simulink model "N3Z_tonetestError"  (R2014b)
settings: Solver=ode3  SolverMode=SingleTasking  StartTime=0.0  StopTime=1e-4  FixedStep=fpgaclk  RelTol=1e-3
PreLoadFcn:
  | %fpgaclk=1/32.768e6
  | fpgaclk=1/49.162e6
  | 
  | SerialData=[1,zeros(1,11),1,0,0,1]
  | load ../N3workingG/window
  | win=win';  %Go back to using flatter and wider windowed sync function
  | %load ../N3workingG/hanning    %use Hahn window
  | 
  | load ../N3workingG/PREemphasis   %For pre-empasis and deemphasis FIRs
  | 
  | %LUT3=xls2LUT2('../IQI_Qdemod.xls'); LUT3
  | load ../N3workingG/LUT3
  | load ../N3workingG/FIRiq2
  | % xls2LUT
  | 
  | GetProgFiles
  | 
  | PinAssignments    %Get Pin references for TE0722
  | 
  | 
  | 
  | 
  | 
  | %LCD
  | LCDdata=[LCD_D7,LCD_D6,LCD_D5,LCD_D4,LCD_D3,LCD_D2,LCD_D1,LCD_D0] %Note MSB...LSB!
  | LCDctrl=[LCD_E,LCD_RW,LCD_RS];
  | 
  | %for RS232 on pins 3 and 5 of USBB
  | 
  | %BT chip connections for WT12
  | 
  | RX_BT=RXD
  | TX_BT=TXD
  | 
  | RST_BB=RES
  | 
  | %PCMC=PCMC
  | %PCMS=PCMS
  | %PCMI=PCMI
  | %PCMO=PCMO
  | 
  | %Aliases:
  | SRDBT=PCMI
  | STDBT=PCMO
  | SCLK_BT=PCMC
  | SFS_BT=PCMS
  | 
  | %ADC control
  | 
  | %SDOA=SDOA
  | %SDOB=SDOB
  | %SCK=SCK
  | CONV=Csbar
  | CAL=Cal
  | 
  | ADC_G=[ADC_G3,ADC_G2,ADC_G1,ADC_G0]
  | %PD settings hard coded now
  | 
  | %%%%%%
  | TX_LOW=TX_Low
  | ... (+11 lines)
StartFcn:
  | SerialData=[1,zeros(1,11),1,0,0,1]
values from neighbouring files (symbols this model uses):
  ADC_G0 = {'P10'}    [PinAssignments.m]
  ADC_G1 = {'P11'}    [PinAssignments.m]
  ADC_G2 = {'N14'}    [PinAssignments.m]
  ADC_G3 = {'M11'}    [PinAssignments.m]
  Cal = {'L12'}    [PinAssignments.m]
  Csbar = {'M12'}    [PinAssignments.m]
  LCD_D0 = {'J13'}    [PinAssignments.m]
  LCD_D1 = {'J14'}    [PinAssignments.m]
  LCD_D2 = {'F15'}    [PinAssignments.m]
  LCD_D3 = {'H14'}    [PinAssignments.m]
  LCD_D4 = {'G12'}    [PinAssignments.m]
  LCD_D5 = {'L15'}    [PinAssignments.m]
  LCD_D6 = {'M14'}    [PinAssignments.m]
  LCD_D7 = {'K15'}    [PinAssignments.m]
  PCMC = {'H11'}    [PinAssignments.m]
  PCMI = {'H12'}    [PinAssignments.m]
  PCMO = {'N13'}    [PinAssignments.m]
  PCMS = {'M10'}    [PinAssignments.m]
  RES = {'G11'}    [PinAssignments.m]
  RXD = {'H13'}    [PinAssignments.m]
  TX_Low = {'P15'}    [PinAssignments.m]
  TXD = {'P13'}    [PinAssignments.m]
undefined symbols (not defined in the file or in its folder): AXI4, FIRRX, FIRTX, Lite
libraries: xbsIndex_r4 x1238, MyFunctions x43
(part 8 of 9)

== system N3Z_tonetestError/KeyPadinterface/OutputRegister/Subsystem5 ==
  Data : Inport
  PortId : Inport  Port=2
  Write : Inport  Port=3
  Logical : xbsIndex_r4/Logical  logical_function=AND  inputs=2  en=off  latency=0  precision=Full  arith_type=Unsigned  n_bits=8  bin_pt=2  align_bp=on  dbl_ovrd=off  block_type=logical
      settings: xl_area=[1 0 0 1 0 0 0]  block_version=VER_STRING_GOES_HERE
  PortAddress : xbsIndex_r4/Constant  const=3  gui_display_data_type=Fixed-point  arith_type=Unsigned  n_bits=8  bin_pt=0  preci_type=Single  exp_width=8  frac_width=24  explicit_period=on  period=fpgaclk  equ=P=C  opselect=C  inp2=PCIN>>17  opr=+  inp1=P  carry=CIN  dbl_ovrd=off  block_type=constant
      settings: block_version=VER_STRING_GOES_HERE
  Register1 : xbsIndex_r4/Register  init=0  rst=off  en=on  dbl_ovrd=off  block_type=register
      settings: xl_area=[4 8 0 0 0 0 0]  block_version=VER_STRING_GOES_HERE
  Relational1 : xbsIndex_r4/Relational  mode=a=b  op_type=Bool  en=off  latency=0  dbl_ovrd=off  block_type=relational
      settings: xl_area=[2 0 0 4 0 0 0]  block_version=VER_STRING_GOES_HERE
  LatchedData : Outport
  wires:
  Relational1/1 -> Logical/1
  Logical/1 -> Register1/2
  PortAddress/1 -> Relational1/2
  Data/1 -> Register1/1
  PortId/1 -> Relational1/1
  Write/1 -> Logical/2
  Register1/1 -> LatchedData/1

== system N3Z_tonetestError/KeyPadinterface/OutputRegister/Subsystem6 ==
  Data : Inport
  PortId : Inport  Port=2
  Write : Inport  Port=3
  Logical : xbsIndex_r4/Logical  logical_function=AND  inputs=2  en=off  latency=0  precision=Full  arith_type=Unsigned  n_bits=8  bin_pt=2  align_bp=on  dbl_ovrd=off  block_type=logical
      settings: xl_area=[1 0 0 1 0 0 0]  block_version=VER_STRING_GOES_HERE
  PortAddress : xbsIndex_r4/Constant  const=7  gui_display_data_type=Fixed-point  arith_type=Unsigned  n_bits=8  bin_pt=0  preci_type=Single  exp_width=8  frac_width=24  explicit_period=on  period=fpgaclk  equ=P=C  opselect=C  inp2=PCIN>>17  opr=+  inp1=P  carry=CIN  dbl_ovrd=off  block_type=constant
      settings: block_version=VER_STRING_GOES_HERE
  Register1 : xbsIndex_r4/Register  init=151  rst=off  en=on  dbl_ovrd=off  block_type=register
      settings: xl_area=[4 8 0 0 0 0 0]  block_version=VER_STRING_GOES_HERE
  Relational1 : xbsIndex_r4/Relational  mode=a=b  op_type=Bool  en=off  latency=0  dbl_ovrd=off  block_type=relational
      settings: xl_area=[2 0 0 4 0 0 0]  block_version=VER_STRING_GOES_HERE
  LatchedData : Outport
  strobe : Outport  Port=2
  wires:
  Relational1/1 -> Logical/1
  Logical/1 -> Register1/2, strobe/1
  PortAddress/1 -> Relational1/2
  Data/1 -> Register1/1
  PortId/1 -> Relational1/1
  Write/1 -> Logical/2
  Register1/1 -> LatchedData/1

== system N3Z_tonetestError/KeyPadinterface/OutputRegister/Subsystem7 ==
  Data : Inport
  PortId : Inport  Port=2
  Write : Inport  Port=3
  Logical : xbsIndex_r4/Logical  logical_function=AND  inputs=2  en=off  latency=0  precision=Full  arith_type=Unsigned  n_bits=8  bin_pt=2  align_bp=on  dbl_ovrd=off  block_type=logical
      settings: xl_area=[1 0 0 1 0 0 0]  block_version=VER_STRING_GOES_HERE
  PortAddress : xbsIndex_r4/Constant  const=9  gui_display_data_type=Fixed-point  arith_type=Unsigned  n_bits=8  bin_pt=0  preci_type=Single  exp_width=8  frac_width=24  explicit_period=on  period=fpgaclk  equ=P=C  opselect=C  inp2=PCIN>>17  opr=+  inp1=P  carry=CIN  dbl_ovrd=off  block_type=constant
      settings: block_version=VER_STRING_GOES_HERE
  Register1 : xbsIndex_r4/Register  init=0  rst=off  en=on  dbl_ovrd=off  block_type=register
      settings: xl_area=[4 8 0 0 0 0 0]  block_version=VER_STRING_GOES_HERE
  Relational1 : xbsIndex_r4/Relational  mode=a=b  op_type=Bool  en=off  latency=0  dbl_ovrd=off  block_type=relational
      settings: xl_area=[2 0 0 4 0 0 0]  block_version=VER_STRING_GOES_HERE
  LatchedData : Outport
  strobe : Outport  Port=2
  wires:
  Relational1/1 -> Logical/1
  Logical/1 -> Register1/2, strobe/1
  PortAddress/1 -> Relational1/2
  Data/1 -> Register1/1
  PortId/1 -> Relational1/1
  Write/1 -> Logical/2
  Register1/1 -> LatchedData/1

== system N3Z_tonetestError/KeyPadinterface/OutputRegister/Subsystem8 ==
  Data : Inport
  PortId : Inport  Port=2
  Write : Inport  Port=3
  Logical : xbsIndex_r4/Logical  logical_function=AND  inputs=2  en=off  latency=0  precision=Full  arith_type=Unsigned  n_bits=8  bin_pt=2  align_bp=on  dbl_ovrd=off  block_type=logical
      settings: xl_area=[1 0 0 1 0 0 0]  block_version=VER_STRING_GOES_HERE
  PortAddress : xbsIndex_r4/Constant  const=8  gui_display_data_type=Fixed-point  arith_type=Unsigned  n_bits=8  bin_pt=0  preci_type=Single  exp_width=8  frac_width=24  explicit_period=on  period=fpgaclk  equ=P=C  opselect=C  inp2=PCIN>>17  opr=+  inp1=P  carry=CIN  dbl_ovrd=off  block_type=constant
      settings: block_version=VER_STRING_GOES_HERE
  Register1 : xbsIndex_r4/Register  init=0  rst=off  en=on  dbl_ovrd=off  block_type=register
      settings: xl_area=[4 8 0 0 0 0 0]  block_version=VER_STRING_GOES_HERE
  Relational1 : xbsIndex_r4/Relational  mode=a=b  op_type=Bool  en=off  latency=0  dbl_ovrd=off  block_type=relational
      settings: xl_area=[2 0 0 4 0 0 0]  block_version=VER_STRING_GOES_HERE
  LatchedData : Outport
  wires:
  Relational1/1 -> Logical/1
  Logical/1 -> Register1/2
  PortAddress/1 -> Relational1/2
  Data/1 -> Register1/1
  PortId/1 -> Relational1/1
  Write/1 -> Logical/2
  Register1/1 -> LatchedData/1

== system N3Z_tonetestError/KeyPadinterface/OutputRegister/Subsystem9 ==
  Data : Inport
  PortId : Inport  Port=2
  Write : Inport  Port=3
  Logical : xbsIndex_r4/Logical  logical_function=AND  inputs=2  en=off  latency=0  precision=Full  arith_type=Unsigned  n_bits=8  bin_pt=2  align_bp=on  dbl_ovrd=off  block_type=logical
      settings: xl_area=[1 0 0 1 0 0 0]  block_version=VER_STRING_GOES_HERE
  PortAddress : xbsIndex_r4/Constant  const=10  gui_display_data_type=Fixed-point  arith_type=Unsigned  n_bits=8  bin_pt=0  preci_type=Single  exp_width=8  frac_width=24  explicit_period=on  period=fpgaclk  equ=P=C  opselect=C  inp2=PCIN>>17  opr=+  inp1=P  carry=CIN  dbl_ovrd=off  block_type=constant
      settings: block_version=VER_STRING_GOES_HERE
  Register1 : xbsIndex_r4/Register  init=floor(30022/256)  rst=off  en=on  dbl_ovrd=off  block_type=register
      settings: xl_area=[4 8 0 0 0 0 0]  block_version=VER_STRING_GOES_HERE
  Relational1 : xbsIndex_r4/Relational  mode=a=b  op_type=Bool  en=off  latency=0  dbl_ovrd=off  block_type=relational
      settings: xl_area=[2 0 0 4 0 0 0]  block_version=VER_STRING_GOES_HERE
  LatchedData : Outport
  wires:
  Relational1/1 -> Logical/1
  Logical/1 -> Register1/2
  PortAddress/1 -> Relational1/2
  Data/1 -> Register1/1
  PortId/1 -> Relational1/1
  Write/1 -> Logical/2
  Register1/1 -> LatchedData/1

== system N3Z_tonetestError/LoranPulsedetect/LranPass/Eighth ==
  note: Assumes one bit already added to left by previous adder so Shifts right 2 and sign extends
  In1 : Inport
  Concat : xbsIndex_r4/Concat  num_inputs=3  dbl_ovrd=off  block_type=concat
      settings: block_version=12.2
  Reinterpret : xbsIndex_r4/Reinterpret  force_arith_type=on  arith_type="Signed  (2's comp)"  force_bin_pt=off  bin_pt=0  block_type=reinterpret
      settings: infoedit="Changes signal type without altering the binary representation.   You can changed the signal between signed and unsigned, and relocate the binary point.<br><br>Hardware notes: In hardware this block costs nothing.<br><br>Example:  Suppose the input is 6 bits wide, signed, with 2 fractional bits, and the output is forced to unsigned with 0 fractional bits.  Then an input of -2.0 (1110.00 in binary 2's complement) becomes an output of 56 (111000 in binary)."  block_version=12.2
  Slice1 : xbsIndex_r4/Slice  nbits=6  boolean_output=off  mode=Upper Bit Location + Width  bit1=0  base1=MSB of Input  bit0=0  base0=LSB of Input  dbl_ovrd=off  block_type=slice
      settings: block_version=12.2
  Slice2 : xbsIndex_r4/Slice  nbits=1  boolean_output=off  mode=Upper Bit Location + Width  bit1=0  base1=MSB of Input  bit0=0  base0=LSB of Input  dbl_ovrd=off  block_type=slice
      settings: block_version=12.2
  Out1 : Outport
  wires:
  Slice2/1 -> Concat/1, Concat/2
  Slice1/1 -> Concat/3
  In1/1 -> Slice2/1, Slice1/1
  Concat/1 -> Reinterpret/1
  Reinterpret/1 -> Out1/1

== system N3Z_tonetestError/LoranPulsedetect/LranPass/Half ==
  note: Assumes already gained one bit to left
  In1 : Inport
  Reinterpret : xbsIndex_r4/Reinterpret  force_arith_type=on  arith_type="Signed  (2's comp)"  force_bin_pt=off  bin_pt=0  block_type=reinterpret
      settings: infoedit="Changes signal type without altering the binary representation.   You can changed the signal between signed and unsigned, and relocate the binary point.<br><br>Hardware notes: In hardware this block costs nothing.<br><br>Example:  Suppose the input is 6 bits wide, signed, with 2 fractional bits, and the output is forced to unsigned with 0 fractional bits.  Then an input of -2.0 (1110.00 in binary 2's complement) becomes an output of 56 (111000 in binary)."  block_version=12.2
  Slice1 : xbsIndex_r4/Slice  nbits=8  boolean_output=off  mode=Upper Bit Location + Width  bit1=0  base1=MSB of Input  bit0=0  base0=LSB of Input  dbl_ovrd=off  block_type=slice
      settings: block_version=12.2
  Out1 : Outport
  wires:
  In1/1 -> Slice1/1
  Slice1/1 -> Reinterpret/1
  Reinterpret/1 -> Out1/1

== system N3Z_tonetestError/LoranPulsedetect/LranPass/Half1 ==
  note: Assumes already gained one bit to left
  In1 : Inport
  Reinterpret : xbsIndex_r4/Reinterpret  force_arith_type=on  arith_type="Signed  (2's comp)"  force_bin_pt=off  bin_pt=0  block_type=reinterpret
      settings: infoedit="Changes signal type without altering the binary representation.   You can changed the signal between signed and unsigned, and relocate the binary point.<br><br>Hardware notes: In hardware this block costs nothing.<br><br>Example:  Suppose the input is 6 bits wide, signed, with 2 fractional bits, and the output is forced to unsigned with 0 fractional bits.  Then an input of -2.0 (1110.00 in binary 2's complement) becomes an output of 56 (111000 in binary)."  block_version=12.2
  Slice1 : xbsIndex_r4/Slice  nbits=8  boolean_output=off  mode=Upper Bit Location + Width  bit1=0  base1=MSB of Input  bit0=0  base0=LSB of Input  dbl_ovrd=off  block_type=slice
      settings: block_version=12.2
  Out1 : Outport
  wires:
  In1/1 -> Slice1/1
  Slice1/1 -> Reinterpret/1
  Reinterpret/1 -> Out1/1

== system N3Z_tonetestError/LoranPulsedetect/LranPass/Quarter ==
  note: Assumes already gained 1 bit soShifts right 1 and sign extends
  In1 : Inport
  Concat : xbsIndex_r4/Concat  num_inputs=2  dbl_ovrd=off  block_type=concat
      settings: block_version=12.2
  Reinterpret : xbsIndex_r4/Reinterpret  force_arith_type=on  arith_type="Signed  (2's comp)"  force_bin_pt=off  bin_pt=0  block_type=reinterpret
      settings: infoedit="Changes signal type without altering the binary representation.   You can changed the signal between signed and unsigned, and relocate the binary point.<br><br>Hardware notes: In hardware this block costs nothing.<br><br>Example:  Suppose the input is 6 bits wide, signed, with 2 fractional bits, and the output is forced to unsigned with 0 fractional bits.  Then an input of -2.0 (1110.00 in binary 2's complement) becomes an output of 56 (111000 in binary)."  block_version=12.2
  Slice1 : xbsIndex_r4/Slice  nbits=7  boolean_output=off  mode=Upper Bit Location + Width  bit1=0  base1=MSB of Input  bit0=0  base0=LSB of Input  dbl_ovrd=off  block_type=slice
      settings: block_version=12.2
  Slice2 : xbsIndex_r4/Slice  nbits=1  boolean_output=off  mode=Upper Bit Location + Width  bit1=0  base1=MSB of Input  bit0=0  base0=LSB of Input  dbl_ovrd=off  block_type=slice
      settings: block_version=12.2
  Out1 : Outport
  wires:
  Slice2/1 -> Concat/1
  Slice1/1 -> Concat/2
  In1/1 -> Slice2/1, Slice1/1
  Concat/1 -> Reinterpret/1
  Reinterpret/1 -> Out1/1

== system N3Z_tonetestError/LoranPulsedetect/LranPass/Quarter2 ==
  note: Assumes already gained 1 bit soShifts right 1 and sign extends
  In1 : Inport
  Concat : xbsIndex_r4/Concat  num_inputs=2  dbl_ovrd=off  block_type=concat
      settings: block_version=12.2
  Reinterpret : xbsIndex_r4/Reinterpret  force_arith_type=on  arith_type="Signed  (2's comp)"  force_bin_pt=off  bin_pt=0  block_type=reinterpret
      settings: infoedit="Changes signal type without altering the binary representation.   You can changed the signal between signed and unsigned, and relocate the binary point.<br><br>Hardware notes: In hardware this block costs nothing.<br><br>Example:  Suppose the input is 6 bits wide, signed, with 2 fractional bits, and the output is forced to unsigned with 0 fractional bits.  Then an input of -2.0 (1110.00 in binary 2's complement) becomes an output of 56 (111000 in binary)."  block_version=12.2
  Slice1 : xbsIndex_r4/Slice  nbits=7  boolean_output=off  mode=Upper Bit Location + Width  bit1=0  base1=MSB of Input  bit0=0  base0=LSB of Input  dbl_ovrd=off  block_type=slice
      settings: block_version=12.2
  Slice2 : xbsIndex_r4/Slice  nbits=1  boolean_output=off  mode=Upper Bit Location + Width  bit1=0  base1=MSB of Input  bit0=0  base0=LSB of Input  dbl_ovrd=off  block_type=slice
      settings: block_version=12.2
  Out1 : Outport
  wires:
  Slice2/1 -> Concat/1
  Slice1/1 -> Concat/2
  In1/1 -> Slice2/1, Slice1/1
  Concat/1 -> Reinterpret/1
  Reinterpret/1 -> Out1/1

== system N3Z_tonetestError/ToneDetect/OutputRegister/Subsystem1 ==
  Data : Inport
  PortId : Inport  Port=2
  Write : Inport  Port=3
  Logical : xbsIndex_r4/Logical  logical_function=AND  inputs=2  en=off  latency=0  precision=Full  arith_type=Unsigned  n_bits=8  bin_pt=2  align_bp=on  dbl_ovrd=off  block_type=logical
      settings: xl_area=[1 0 0 1 0 0 0]  block_version=VER_STRING_GOES_HERE
  PortAddress : xbsIndex_r4/Constant  const=3  gui_display_data_type=Fixed-point  arith_type=Unsigned  n_bits=8  bin_pt=0  preci_type=Single  exp_width=8  frac_width=24  explicit_period=on  period=fpgaclk  equ=P=C  opselect=C  inp2=PCIN>>17  opr=+  inp1=P  carry=CIN  dbl_ovrd=off  block_type=constant
      settings: block_version=VER_STRING_GOES_HERE
  Register1 : xbsIndex_r4/Register  init=0  rst=off  en=on  dbl_ovrd=off  block_type=register
      settings: xl_area=[4 8 0 0 0 0 0]  block_version=VER_STRING_GOES_HERE
  Relational1 : xbsIndex_r4/Relational  mode=a=b  op_type=Bool  en=off  latency=0  dbl_ovrd=off  block_type=relational
      settings: xl_area=[2 0 0 4 0 0 0]  block_version=VER_STRING_GOES_HERE
  LatchedData : Outport
  Strobe : Outport  Port=2
  wires:
  Relational1/1 -> Logical/1
  Logical/1 -> Register1/2, Strobe/1
  PortAddress/1 -> Relational1/2
  Data/1 -> Register1/1
  PortId/1 -> Relational1/1
  Write/1 -> Logical/2
  Register1/1 -> LatchedData/1

== system N3Z_tonetestError/ToneDetect/OutputRegister/Subsystem10 ==
  Data : Inport
  PortId : Inport  Port=2
  Write : Inport  Port=3
  Logical : xbsIndex_r4/Logical  logical_function=AND  inputs=2  en=off  latency=0  precision=Full  arith_type=Unsigned  n_bits=8  bin_pt=2  align_bp=on  dbl_ovrd=off  block_type=logical
      settings: xl_area=[1 0 0 1 0 0 0]  block_version=VER_STRING_GOES_HERE
  PortAddress : xbsIndex_r4/Constant  const=14  gui_display_data_type=Fixed-point  arith_type=Unsigned  n_bits=8  bin_pt=0  preci_type=Single  exp_width=8  frac_width=24  explicit_period=on  period=fpgaclk  equ=P=C  opselect=C  inp2=PCIN>>17  opr=+  inp1=P  carry=CIN  dbl_ovrd=off  block_type=constant
      settings: block_version=VER_STRING_GOES_HERE
  Register1 : xbsIndex_r4/Register  init=0  rst=off  en=on  dbl_ovrd=off  block_type=register
      settings: xl_area=[4 8 0 0 0 0 0]  block_version=VER_STRING_GOES_HERE
  Relational1 : xbsIndex_r4/Relational  mode=a=b  op_type=Bool  en=off  latency=0  dbl_ovrd=off  block_type=relational
      settings: xl_area=[2 0 0 4 0 0 0]  block_version=VER_STRING_GOES_HERE
  LatchedData : Outport
  Strobe : Outport  Port=2
  wires:
  Relational1/1 -> Logical/1
  Logical/1 -> Register1/2, Strobe/1
  PortAddress/1 -> Relational1/2
  Data/1 -> Register1/1
  PortId/1 -> Relational1/1
  Write/1 -> Logical/2
  Register1/1 -> LatchedData/1

== system N3Z_tonetestError/ToneDetect/OutputRegister/Subsystem11 ==
  Data : Inport
  PortId : Inport  Port=2
  Write : Inport  Port=3
  Logical : xbsIndex_r4/Logical  logical_function=AND  inputs=2  en=off  latency=0  precision=Full  arith_type=Unsigned  n_bits=8  bin_pt=2  align_bp=on  dbl_ovrd=off  block_type=logical
      settings: xl_area=[1 0 0 1 0 0 0]  block_version=VER_STRING_GOES_HERE
  PortAddress : xbsIndex_r4/Constant  const=19  gui_display_data_type=Fixed-point  arith_type=Unsigned  n_bits=8  bin_pt=0  preci_type=Single  exp_width=8  frac_width=24  explicit_period=on  period=fpgaclk  equ=P=C  opselect=C  inp2=PCIN>>17  opr=+  inp1=P  carry=CIN  dbl_ovrd=off  block_type=constant
      settings: block_version=VER_STRING_GOES_HERE
  Register1 : xbsIndex_r4/Register  init=0  rst=off  en=on  dbl_ovrd=off  block_type=register
      settings: xl_area=[4 8 0 0 0 0 0]  block_version=VER_STRING_GOES_HERE
  Relational1 : xbsIndex_r4/Relational  mode=a=b  op_type=Bool  en=off  latency=0  dbl_ovrd=off  block_type=relational
      settings: xl_area=[2 0 0 4 0 0 0]  block_version=VER_STRING_GOES_HERE
  LatchedData : Outport
  Strobe : Outport  Port=2
  wires:
  Relational1/1 -> Logical/1
  Logical/1 -> Register1/2, Strobe/1
  PortAddress/1 -> Relational1/2
  Data/1 -> Register1/1
  PortId/1 -> Relational1/1
  Write/1 -> Logical/2
  Register1/1 -> LatchedData/1

== system N3Z_tonetestError/ToneDetect/OutputRegister/Subsystem12 ==
  Data : Inport
  PortId : Inport  Port=2
  Write : Inport  Port=3
  Logical : xbsIndex_r4/Logical  logical_function=AND  inputs=2  en=off  latency=0  precision=Full  arith_type=Unsigned  n_bits=8  bin_pt=2  align_bp=on  dbl_ovrd=off  block_type=logical
      settings: xl_area=[1 0 0 1 0 0 0]  block_version=VER_STRING_GOES_HERE
  PortAddress : xbsIndex_r4/Constant  const=24  gui_display_data_type=Fixed-point  arith_type=Unsigned  n_bits=8  bin_pt=0  preci_type=Single  exp_width=8  frac_width=24  explicit_period=on  period=fpgaclk  equ=P=C  opselect=C  inp2=PCIN>>17  opr=+  inp1=P  carry=CIN  dbl_ovrd=off  block_type=constant
      settings: block_version=VER_STRING_GOES_HERE
  Register1 : xbsIndex_r4/Register  init=0  rst=off  en=on  dbl_ovrd=off  block_type=register
      settings: xl_area=[4 8 0 0 0 0 0]  block_version=VER_STRING_GOES_HERE
  Relational1 : xbsIndex_r4/Relational  mode=a=b  op_type=Bool  en=off  latency=0  dbl_ovrd=off  block_type=relational
      settings: xl_area=[2 0 0 4 0 0 0]  block_version=VER_STRING_GOES_HERE
  LatchedData : Outport
  Strobe : Outport  Port=2
  wires:
  Relational1/1 -> Logical/1
  Logical/1 -> Register1/2, Strobe/1
  PortAddress/1 -> Relational1/2
  Data/1 -> Register1/1
  PortId/1 -> Relational1/1
  Write/1 -> Logical/2
  Register1/1 -> LatchedData/1

== system N3Z_tonetestError/ToneDetect/OutputRegister/Subsystem13 ==
  Data : Inport
  PortId : Inport  Port=2
  Write : Inport  Port=3
  Logical : xbsIndex_r4/Logical  logical_function=AND  inputs=2  en=off  latency=0  precision=Full  arith_type=Unsigned  n_bits=8  bin_pt=2  align_bp=on  dbl_ovrd=off  block_type=logical
      settings: xl_area=[1 0 0 1 0 0 0]  block_version=VER_STRING_GOES_HERE
  PortAddress : xbsIndex_r4/Constant  const=12  gui_display_data_type=Fixed-point  arith_type=Unsigned  n_bits=8  bin_pt=0  preci_type=Single  exp_width=8  frac_width=24  explicit_period=on  period=fpgaclk  equ=P=C  opselect=C  inp2=PCIN>>17  opr=+  inp1=P  carry=CIN  dbl_ovrd=off  block_type=constant
      settings: block_version=VER_STRING_GOES_HERE
  Register1 : xbsIndex_r4/Register  init=0  rst=off  en=on  dbl_ovrd=off  block_type=register
      settings: xl_area=[4 8 0 0 0 0 0]  block_version=VER_STRING_GOES_HERE
  Relational1 : xbsIndex_r4/Relational  mode=a=b  op_type=Bool  en=off  latency=0  dbl_ovrd=off  block_type=relational
      settings: xl_area=[2 0 0 4 0 0 0]  block_version=VER_STRING_GOES_HERE
  LatchedData : Outport
  Strobe : Outport  Port=2
  wires:
  Relational1/1 -> Logical/1
  Logical/1 -> Register1/2, Strobe/1
  PortAddress/1 -> Relational1/2
  Data/1 -> Register1/1
  PortId/1 -> Relational1/1
  Write/1 -> Logical/2
  Register1/1 -> LatchedData/1

== system N3Z_tonetestError/ToneDetect/OutputRegister/Subsystem14 ==
  Data : Inport
  PortId : Inport  Port=2
  Write : Inport  Port=3
  Logical : xbsIndex_r4/Logical  logical_function=AND  inputs=2  en=off  latency=0  precision=Full  arith_type=Unsigned  n_bits=8  bin_pt=2  align_bp=on  dbl_ovrd=off  block_type=logical
      settings: xl_area=[1 0 0 1 0 0 0]  block_version=VER_STRING_GOES_HERE
  PortAddress : xbsIndex_r4/Constant  const=17  gui_display_data_type=Fixed-point  arith_type=Unsigned  n_bits=8  bin_pt=0  preci_type=Single  exp_width=8  frac_width=24  explicit_period=on  period=fpgaclk  equ=P=C  opselect=C  inp2=PCIN>>17  opr=+  inp1=P  carry=CIN  dbl_ovrd=off  block_type=constant
      settings: block_version=VER_STRING_GOES_HERE
  Register1 : xbsIndex_r4/Register  init=0  rst=off  en=on  dbl_ovrd=off  block_type=register
      settings: xl_area=[4 8 0 0 0 0 0]  block_version=VER_STRING_GOES_HERE
  Relational1 : xbsIndex_r4/Relational  mode=a=b  op_type=Bool  en=off  latency=0  dbl_ovrd=off  block_type=relational
      settings: xl_area=[2 0 0 4 0 0 0]  block_version=VER_STRING_GOES_HERE
  LatchedData : Outport
  Strobe : Outport  Port=2
  wires:
  Relational1/1 -> Logical/1
  Logical/1 -> Register1/2, Strobe/1
  PortAddress/1 -> Relational1/2
  Data/1 -> Register1/1
  PortId/1 -> Relational1/1
  Write/1 -> Logical/2
  Register1/1 -> LatchedData/1

== system N3Z_tonetestError/ToneDetect/OutputRegister/Subsystem15 ==
  Data : Inport
  PortId : Inport  Port=2
  Write : Inport  Port=3
  Logical : xbsIndex_r4/Logical  logical_function=AND  inputs=2  en=off  latency=0  precision=Full  arith_type=Unsigned  n_bits=8  bin_pt=2  align_bp=on  dbl_ovrd=off  block_type=logical
      settings: xl_area=[1 0 0 1 0 0 0]  block_version=VER_STRING_GOES_HERE
  PortAddress : xbsIndex_r4/Constant  const=22  gui_display_data_type=Fixed-point  arith_type=Unsigned  n_bits=8  bin_pt=0  preci_type=Single  exp_width=8  frac_width=24  explicit_period=on  period=fpgaclk  equ=P=C  opselect=C  inp2=PCIN>>17  opr=+  inp1=P  carry=CIN  dbl_ovrd=off  block_type=constant
      settings: block_version=VER_STRING_GOES_HERE
  Register1 : xbsIndex_r4/Register  init=0  rst=off  en=on  dbl_ovrd=off  block_type=register
      settings: xl_area=[4 8 0 0 0 0 0]  block_version=VER_STRING_GOES_HERE
  Relational1 : xbsIndex_r4/Relational  mode=a=b  op_type=Bool  en=off  latency=0  dbl_ovrd=off  block_type=relational
      settings: xl_area=[2 0 0 4 0 0 0]  block_version=VER_STRING_GOES_HERE
  LatchedData : Outport
  Strobe : Outport  Port=2
  wires:
  Relational1/1 -> Logical/1
  Logical/1 -> Register1/2, Strobe/1
  PortAddress/1 -> Relational1/2
  Data/1 -> Register1/1
  PortId/1 -> Relational1/1
  Write/1 -> Logical/2
  Register1/1 -> LatchedData/1

== system N3Z_tonetestError/ToneDetect/OutputRegister/Subsystem16 ==
  Data : Inport
  PortId : Inport  Port=2
  Write : Inport  Port=3
  Logical : xbsIndex_r4/Logical  logical_function=AND  inputs=2  en=off  latency=0  precision=Full  arith_type=Unsigned  n_bits=8  bin_pt=2  align_bp=on  dbl_ovrd=off  block_type=logical
      settings: xl_area=[1 0 0 1 0 0 0]  block_version=VER_STRING_GOES_HERE
  PortAddress : xbsIndex_r4/Constant  const=6  gui_display_data_type=Fixed-point  arith_type=Unsigned  n_bits=8  bin_pt=0  preci_type=Single  exp_width=8  frac_width=24  explicit_period=on  period=fpgaclk  equ=P=C  opselect=C  inp2=PCIN>>17  opr=+  inp1=P  carry=CIN  dbl_ovrd=off  block_type=constant
      settings: block_version=VER_STRING_GOES_HERE
  Register1 : xbsIndex_r4/Register  init=0  rst=off  en=on  dbl_ovrd=off  block_type=register
      settings: xl_area=[4 8 0 0 0 0 0]  block_version=VER_STRING_GOES_HERE
  Relational1 : xbsIndex_r4/Relational  mode=a=b  op_type=Bool  en=off  latency=0  dbl_ovrd=off  block_type=relational
      settings: xl_area=[2 0 0 4 0 0 0]  block_version=VER_STRING_GOES_HERE
  LatchedData : Outport
  Strobe : Outport  Port=2
  wires:
  Relational1/1 -> Logical/1
  Logical/1 -> Register1/2, Strobe/1
  PortAddress/1 -> Relational1/2
  Data/1 -> Register1/1
  PortId/1 -> Relational1/1
  Write/1 -> Logical/2
  Register1/1 -> LatchedData/1

== system N3Z_tonetestError/ToneDetect/OutputRegister/Subsystem17 ==
  Data : Inport
  PortId : Inport  Port=2
  Write : Inport  Port=3
  Logical : xbsIndex_r4/Logical  logical_function=AND  inputs=2  en=off  latency=0  precision=Full  arith_type=Unsigned  n_bits=8  bin_pt=2  align_bp=on  dbl_ovrd=off  block_type=logical
      settings: xl_area=[1 0 0 1 0 0 0]  block_version=VER_STRING_GOES_HERE
  PortAddress : xbsIndex_r4/Constant  const=11  gui_display_data_type=Fixed-point  arith_type=Unsigned  n_bits=8  bin_pt=0  preci_type=Single  exp_width=8  frac_width=24  explicit_period=on  period=fpgaclk  equ=P=C  opselect=C  inp2=PCIN>>17  opr=+  inp1=P  carry=CIN  dbl_ovrd=off  block_type=constant
      settings: block_version=VER_STRING_GOES_HERE
  Register1 : xbsIndex_r4/Register  init=0  rst=off  en=on  dbl_ovrd=off  block_type=register
      settings: xl_area=[4 8 0 0 0 0 0]  block_version=VER_STRING_GOES_HERE
  Relational1 : xbsIndex_r4/Relational  mode=a=b  op_type=Bool  en=off  latency=0  dbl_ovrd=off  block_type=relational
      settings: xl_area=[2 0 0 4 0 0 0]  block_version=VER_STRING_GOES_HERE
  LatchedData : Outport
  Strobe : Outport  Port=2
  wires:
  Relational1/1 -> Logical/1
  Logical/1 -> Register1/2, Strobe/1
  PortAddress/1 -> Relational1/2
  Data/1 -> Register1/1
  PortId/1 -> Relational1/1
  Write/1 -> Logical/2
  Register1/1 -> LatchedData/1

== system N3Z_tonetestError/ToneDetect/OutputRegister/Subsystem18 ==
  Data : Inport
  PortId : Inport  Port=2
  Write : Inport  Port=3
  Logical : xbsIndex_r4/Logical  logical_function=AND  inputs=2  en=off  latency=0  precision=Full  arith_type=Unsigned  n_bits=8  bin_pt=2  align_bp=on  dbl_ovrd=off  block_type=logical
      settings: xl_area=[1 0 0 1 0 0 0]  block_version=VER_STRING_GOES_HERE
  PortAddress : xbsIndex_r4/Constant  const=16  gui_display_data_type=Fixed-point  arith_type=Unsigned  n_bits=8  bin_pt=0  preci_type=Single  exp_width=8  frac_width=24  explicit_period=on  period=fpgaclk  equ=P=C  opselect=C  inp2=PCIN>>17  opr=+  inp1=P  carry=CIN  dbl_ovrd=off  block_type=constant
      settings: block_version=VER_STRING_GOES_HERE
  Register1 : xbsIndex_r4/Register  init=0  rst=off  en=on  dbl_ovrd=off  block_type=register
      settings: xl_area=[4 8 0 0 0 0 0]  block_version=VER_STRING_GOES_HERE
  Relational1 : xbsIndex_r4/Relational  mode=a=b  op_type=Bool  en=off  latency=0  dbl_ovrd=off  block_type=relational
      settings: xl_area=[2 0 0 4 0 0 0]  block_version=VER_STRING_GOES_HERE
  LatchedData : Outport
  Strobe : Outport  Port=2
  wires:
  Relational1/1 -> Logical/1
  Logical/1 -> Register1/2, Strobe/1
  PortAddress/1 -> Relational1/2
  Data/1 -> Register1/1
  PortId/1 -> Relational1/1
  Write/1 -> Logical/2
  Register1/1 -> LatchedData/1

== system N3Z_tonetestError/ToneDetect/OutputRegister/Subsystem19 ==
  Data : Inport
  PortId : Inport  Port=2
  Write : Inport  Port=3
  Logical : xbsIndex_r4/Logical  logical_function=AND  inputs=2  en=off  latency=0  precision=Full  arith_type=Unsigned  n_bits=8  bin_pt=2  align_bp=on  dbl_ovrd=off  block_type=logical
      settings: xl_area=[1 0 0 1 0 0 0]  block_version=VER_STRING_GOES_HERE
  PortAddress : xbsIndex_r4/Constant  const=21  gui_display_data_type=Fixed-point  arith_type=Unsigned  n_bits=8  bin_pt=0  preci_type=Single  exp_width=8  frac_width=24  explicit_period=on  period=fpgaclk  equ=P=C  opselect=C  inp2=PCIN>>17  opr=+  inp1=P  carry=CIN  dbl_ovrd=off  block_type=constant
      settings: block_version=VER_STRING_GOES_HERE
  Register1 : xbsIndex_r4/Register  init=0  rst=off  en=on  dbl_ovrd=off  block_type=register
      settings: xl_area=[4 8 0 0 0 0 0]  block_version=VER_STRING_GOES_HERE
  Relational1 : xbsIndex_r4/Relational  mode=a=b  op_type=Bool  en=off  latency=0  dbl_ovrd=off  block_type=relational
      settings: xl_area=[2 0 0 4 0 0 0]  block_version=VER_STRING_GOES_HERE
  LatchedData : Outport
  Strobe : Outport  Port=2
  wires:
  Relational1/1 -> Logical/1
  Logical/1 -> Register1/2, Strobe/1
  PortAddress/1 -> Relational1/2
  Data/1 -> Register1/1
  PortId/1 -> Relational1/1
  Write/1 -> Logical/2
  Register1/1 -> LatchedData/1

== system N3Z_tonetestError/ToneDetect/OutputRegister/Subsystem2 ==
  Data : Inport
  PortId : Inport  Port=2
  Write : Inport  Port=3
  Logical : xbsIndex_r4/Logical  logical_function=AND  inputs=2  en=off  latency=0  precision=Full  arith_type=Unsigned  n_bits=8  bin_pt=2  align_bp=on  dbl_ovrd=off  block_type=logical
      settings: xl_area=[1 0 0 1 0 0 0]  block_version=VER_STRING_GOES_HERE
  PortAddress : xbsIndex_r4/Constant  const=0  gui_display_data_type=Fixed-point  arith_type=Unsigned  n_bits=8  bin_pt=0  preci_type=Single  exp_width=8  frac_width=24  explicit_period=on  period=fpgaclk  equ=P=C  opselect=C  inp2=PCIN>>17  opr=+  inp1=P  carry=CIN  dbl_ovrd=off  block_type=constant
      settings: block_version=VER_STRING_GOES_HERE
  Register1 : xbsIndex_r4/Register  init=0  rst=off  en=on  dbl_ovrd=off  block_type=register
      settings: xl_area=[4 8 0 0 0 0 0]  block_version=VER_STRING_GOES_HERE
  Relational1 : xbsIndex_r4/Relational  mode=a=b  op_type=Bool  en=off  latency=0  dbl_ovrd=off  block_type=relational
      settings: xl_area=[2 0 0 4 0 0 0]  block_version=VER_STRING_GOES_HERE
  LatchedData : Outport
  Strobe : Outport  Port=2
  wires:
  Relational1/1 -> Logical/1
  Logical/1 -> Register1/2, Strobe/1
  PortAddress/1 -> Relational1/2
  Data/1 -> Register1/1
  PortId/1 -> Relational1/1
  Write/1 -> Logical/2
  Register1/1 -> LatchedData/1

== system N3Z_tonetestError/ToneDetect/OutputRegister/Subsystem20 ==
  Data : Inport
  PortId : Inport  Port=2
  Write : Inport  Port=3
  Logical : xbsIndex_r4/Logical  logical_function=AND  inputs=2  en=off  latency=0  precision=Full  arith_type=Unsigned  n_bits=8  bin_pt=2  align_bp=on  dbl_ovrd=off  block_type=logical
      settings: xl_area=[1 0 0 1 0 0 0]  block_version=VER_STRING_GOES_HERE
  PortAddress : xbsIndex_r4/Constant  const=7  gui_display_data_type=Fixed-point  arith_type=Unsigned  n_bits=8  bin_pt=0  preci_type=Single  exp_width=8  frac_width=24  explicit_period=on  period=fpgaclk  equ=P=C  opselect=C  inp2=PCIN>>17  opr=+  inp1=P  carry=CIN  dbl_ovrd=off  block_type=constant
      settings: block_version=VER_STRING_GOES_HERE
  Register1 : xbsIndex_r4/Register  init=0  rst=off  en=on  dbl_ovrd=off  block_type=register
      settings: xl_area=[4 8 0 0 0 0 0]  block_version=VER_STRING_GOES_HERE
  Relational1 : xbsIndex_r4/Relational  mode=a=b  op_type=Bool  en=off  latency=0  dbl_ovrd=off  block_type=relational
      settings: xl_area=[2 0 0 4 0 0 0]  block_version=VER_STRING_GOES_HERE
  LatchedData : Outport
  Strobe : Outport  Port=2
  wires:
  Relational1/1 -> Logical/1
  Logical/1 -> Register1/2, Strobe/1
  PortAddress/1 -> Relational1/2
  Data/1 -> Register1/1
  PortId/1 -> Relational1/1
  Write/1 -> Logical/2
  Register1/1 -> LatchedData/1

== system N3Z_tonetestError/ToneDetect/OutputRegister/Subsystem25 ==
  Data : Inport
  PortId : Inport  Port=2
  Write : Inport  Port=3
  Logical : xbsIndex_r4/Logical  logical_function=AND  inputs=2  en=off  latency=0  precision=Full  arith_type=Unsigned  n_bits=8  bin_pt=2  align_bp=on  dbl_ovrd=off  block_type=logical
      settings: xl_area=[1 0 0 1 0 0 0]  block_version=VER_STRING_GOES_HERE
  PortAddress : xbsIndex_r4/Constant  const=25  gui_display_data_type=Fixed-point  arith_type=Unsigned  n_bits=8  bin_pt=0  preci_type=Single  exp_width=8  frac_width=24  explicit_period=on  period=fpgaclk  equ=P=C  opselect=C  inp2=PCIN>>17  opr=+  inp1=P  carry=CIN  dbl_ovrd=off  block_type=constant
      settings: block_version=VER_STRING_GOES_HERE
  Register1 : xbsIndex_r4/Register  init=0  rst=off  en=on  dbl_ovrd=off  block_type=register
      settings: xl_area=[4 8 0 0 0 0 0]  block_version=VER_STRING_GOES_HERE
  Relational1 : xbsIndex_r4/Relational  mode=a=b  op_type=Bool  en=off  latency=0  dbl_ovrd=off  block_type=relational
      settings: xl_area=[2 0 0 4 0 0 0]  block_version=VER_STRING_GOES_HERE
  LatchedData : Outport
  Strobe : Outport  Port=2
  wires:
  Relational1/1 -> Logical/1
  Logical/1 -> Register1/2, Strobe/1
  PortAddress/1 -> Relational1/2
  Data/1 -> Register1/1
  PortId/1 -> Relational1/1
  Write/1 -> Logical/2
  Register1/1 -> LatchedData/1

== system N3Z_tonetestError/ToneDetect/OutputRegister/Subsystem26 ==
  Data : Inport
  PortId : Inport  Port=2
  Write : Inport  Port=3
  Logical : xbsIndex_r4/Logical  logical_function=AND  inputs=2  en=off  latency=0  precision=Full  arith_type=Unsigned  n_bits=8  bin_pt=2  align_bp=on  dbl_ovrd=off  block_type=logical
      settings: xl_area=[1 0 0 1 0 0 0]  block_version=VER_STRING_GOES_HERE
  PortAddress : xbsIndex_r4/Constant  const=26  gui_display_data_type=Fixed-point  arith_type=Unsigned  n_bits=8  bin_pt=0  preci_type=Single  exp_width=8  frac_width=24  explicit_period=on  period=fpgaclk  equ=P=C  opselect=C  inp2=PCIN>>17  opr=+  inp1=P  carry=CIN  dbl_ovrd=off  block_type=constant
      settings: block_version=VER_STRING_GOES_HERE
  Register1 : xbsIndex_r4/Register  init=1  rst=off  en=on  dbl_ovrd=off  block_type=register
      settings: xl_area=[4 8 0 0 0 0 0]  block_version=VER_STRING_GOES_HERE
  Relational1 : xbsIndex_r4/Relational  mode=a=b  op_type=Bool  en=off  latency=0  dbl_ovrd=off  block_type=relational
      settings: xl_area=[2 0 0 4 0 0 0]  block_version=VER_STRING_GOES_HERE
  LatchedData : Outport
  Strobe : Outport  Port=2
  wires:
  Relational1/1 -> Logical/1
  Logical/1 -> Register1/2, Strobe/1
  PortAddress/1 -> Relational1/2
  Data/1 -> Register1/1
  PortId/1 -> Relational1/1
  Write/1 -> Logical/2
  Register1/1 -> LatchedData/1

== system N3Z_tonetestError/ToneDetect/OutputRegister/Subsystem3 ==
  Data : Inport
  PortId : Inport  Port=2
  Write : Inport  Port=3
  Logical : xbsIndex_r4/Logical  logical_function=AND  inputs=2  en=off  latency=0  precision=Full  arith_type=Unsigned  n_bits=8  bin_pt=2  align_bp=on  dbl_ovrd=off  block_type=logical
      settings: xl_area=[1 0 0 1 0 0 0]  block_version=VER_STRING_GOES_HERE
  PortAddress : xbsIndex_r4/Constant  const=1  gui_display_data_type=Fixed-point  arith_type=Unsigned  n_bits=8  bin_pt=0  preci_type=Single  exp_width=8  frac_width=24  explicit_period=on  period=fpgaclk  equ=P=C  opselect=C  inp2=PCIN>>17  opr=+  inp1=P  carry=CIN  dbl_ovrd=off  block_type=constant
      settings: block_version=VER_STRING_GOES_HERE
  Register1 : xbsIndex_r4/Register  init=0  rst=off  en=on  dbl_ovrd=off  block_type=register
      settings: xl_area=[4 8 0 0 0 0 0]  block_version=VER_STRING_GOES_HERE
  Relational1 : xbsIndex_r4/Relational  mode=a=b  op_type=Bool  en=off  latency=0  dbl_ovrd=off  block_type=relational
      settings: xl_area=[2 0 0 4 0 0 0]  block_version=VER_STRING_GOES_HERE
  LatchedData : Outport
  Strobe : Outport  Port=2
  wires:
  Relational1/1 -> Logical/1
  Logical/1 -> Strobe/1, Register1/2
  PortAddress/1 -> Relational1/2
  Data/1 -> Register1/1
  PortId/1 -> Relational1/1
  Write/1 -> Logical/2
  Register1/1 -> LatchedData/1

== system N3Z_tonetestError/ToneDetect/OutputRegister/Subsystem4 ==
  Data : Inport
  PortId : Inport  Port=2
  Write : Inport  Port=3
  Logical : xbsIndex_r4/Logical  logical_function=AND  inputs=2  en=off  latency=0  precision=Full  arith_type=Unsigned  n_bits=8  bin_pt=2  align_bp=on  dbl_ovrd=off  block_type=logical
      settings: xl_area=[1 0 0 1 0 0 0]  block_version=VER_STRING_GOES_HERE
  PortAddress : xbsIndex_r4/Constant  const=2  gui_display_data_type=Fixed-point  arith_type=Unsigned  n_bits=8  bin_pt=0  preci_type=Single  exp_width=8  frac_width=24  explicit_period=on  period=fpgaclk  equ=P=C  opselect=C  inp2=PCIN>>17  opr=+  inp1=P  carry=CIN  dbl_ovrd=off  block_type=constant
      settings: block_version=VER_STRING_GOES_HERE
  Register1 : xbsIndex_r4/Register  init=0  rst=off  en=on  dbl_ovrd=off  block_type=register
      settings: xl_area=[4 8 0 0 0 0 0]  block_version=VER_STRING_GOES_HERE
  Relational1 : xbsIndex_r4/Relational  mode=a=b  op_type=Bool  en=off  latency=0  dbl_ovrd=off  block_type=relational
      settings: xl_area=[2 0 0 4 0 0 0]  block_version=VER_STRING_GOES_HERE
  LatchedData : Outport
  wires:
  Relational1/1 -> Logical/1
  Logical/1 -> Register1/2
  PortAddress/1 -> Relational1/2
  Data/1 -> Register1/1
  PortId/1 -> Relational1/1
  Write/1 -> Logical/2
  Register1/1 -> LatchedData/1

== system N3Z_tonetestError/ToneDetect/OutputRegister/Subsystem5 ==
  Data : Inport
  PortId : Inport  Port=2
  Write : Inport  Port=3
  Logical : xbsIndex_r4/Logical  logical_function=AND  inputs=2  en=off  latency=0  precision=Full  arith_type=Unsigned  n_bits=8  bin_pt=2  align_bp=on  dbl_ovrd=off  block_type=logical
      settings: xl_area=[1 0 0 1 0 0 0]  block_version=VER_STRING_GOES_HERE
  PortAddress : xbsIndex_r4/Constant  const=8  gui_display_data_type=Fixed-point  arith_type=Unsigned  n_bits=8  bin_pt=0  preci_type=Single  exp_width=8  frac_width=24  explicit_period=on  period=fpgaclk  equ=P=C  opselect=C  inp2=PCIN>>17  opr=+  inp1=P  carry=CIN  dbl_ovrd=off  block_type=constant
      settings: block_version=VER_STRING_GOES_HERE
  Register1 : xbsIndex_r4/Register  init=0  rst=off  en=on  dbl_ovrd=off  block_type=register
      settings: xl_area=[4 8 0 0 0 0 0]  block_version=VER_STRING_GOES_HERE
  Relational1 : xbsIndex_r4/Relational  mode=a=b  op_type=Bool  en=off  latency=0  dbl_ovrd=off  block_type=relational
      settings: xl_area=[2 0 0 4 0 0 0]  block_version=VER_STRING_GOES_HERE
  LatchedData : Outport
  Strobe : Outport  Port=2
  wires:
  Relational1/1 -> Logical/1
  Logical/1 -> Register1/2, Strobe/1
  PortAddress/1 -> Relational1/2
  Data/1 -> Register1/1
  PortId/1 -> Relational1/1
  Write/1 -> Logical/2
  Register1/1 -> LatchedData/1

== system N3Z_tonetestError/ToneDetect/OutputRegister/Subsystem6 ==
  Data : Inport
  PortId : Inport  Port=2
  Write : Inport  Port=3
  Logical : xbsIndex_r4/Logical  logical_function=AND  inputs=2  en=off  latency=0  precision=Full  arith_type=Unsigned  n_bits=8  bin_pt=2  align_bp=on  dbl_ovrd=off  block_type=logical
      settings: xl_area=[1 0 0 1 0 0 0]  block_version=VER_STRING_GOES_HERE
  PortAddress : xbsIndex_r4/Constant  const=13  gui_display_data_type=Fixed-point  arith_type=Unsigned  n_bits=8  bin_pt=0  preci_type=Single  exp_width=8  frac_width=24  explicit_period=on  period=fpgaclk  equ=P=C  opselect=C  inp2=PCIN>>17  opr=+  inp1=P  carry=CIN  dbl_ovrd=off  block_type=constant
      settings: block_version=VER_STRING_GOES_HERE
  Register1 : xbsIndex_r4/Register  init=0  rst=off  en=on  dbl_ovrd=off  block_type=register
      settings: xl_area=[4 8 0 0 0 0 0]  block_version=VER_STRING_GOES_HERE
  Relational1 : xbsIndex_r4/Relational  mode=a=b  op_type=Bool  en=off  latency=0  dbl_ovrd=off  block_type=relational
      settings: xl_area=[2 0 0 4 0 0 0]  block_version=VER_STRING_GOES_HERE
  LatchedData : Outport
  Strobe : Outport  Port=2
  wires:
  Relational1/1 -> Logical/1
  Logical/1 -> Register1/2, Strobe/1
  PortAddress/1 -> Relational1/2
  Data/1 -> Register1/1
  PortId/1 -> Relational1/1
  Write/1 -> Logical/2
  Register1/1 -> LatchedData/1

== system N3Z_tonetestError/ToneDetect/OutputRegister/Subsystem7 ==
  Data : Inport
  PortId : Inport  Port=2
  Write : Inport  Port=3
  Logical : xbsIndex_r4/Logical  logical_function=AND  inputs=2  en=off  latency=0  precision=Full  arith_type=Unsigned  n_bits=8  bin_pt=2  align_bp=on  dbl_ovrd=off  block_type=logical
      settings: xl_area=[1 0 0 1 0 0 0]  block_version=VER_STRING_GOES_HERE
  PortAddress : xbsIndex_r4/Constant  const=18  gui_display_data_type=Fixed-point  arith_type=Unsigned  n_bits=8  bin_pt=0  preci_type=Single  exp_width=8  frac_width=24  explicit_period=on  period=fpgaclk  equ=P=C  opselect=C  inp2=PCIN>>17  opr=+  inp1=P  carry=CIN  dbl_ovrd=off  block_type=constant
      settings: block_version=VER_STRING_GOES_HERE
  Register1 : xbsIndex_r4/Register  init=0  rst=off  en=on  dbl_ovrd=off  block_type=register
      settings: xl_area=[4 8 0 0 0 0 0]  block_version=VER_STRING_GOES_HERE
  Relational1 : xbsIndex_r4/Relational  mode=a=b  op_type=Bool  en=off  latency=0  dbl_ovrd=off  block_type=relational
      settings: xl_area=[2 0 0 4 0 0 0]  block_version=VER_STRING_GOES_HERE
  LatchedData : Outport
  Strobe : Outport  Port=2
  wires:
  Relational1/1 -> Logical/1
  Logical/1 -> Register1/2, Strobe/1
  PortAddress/1 -> Relational1/2
  Data/1 -> Register1/1
  PortId/1 -> Relational1/1
  Write/1 -> Logical/2
  Register1/1 -> LatchedData/1

== system N3Z_tonetestError/ToneDetect/OutputRegister/Subsystem8 ==
  Data : Inport
  PortId : Inport  Port=2
  Write : Inport  Port=3
  Logical : xbsIndex_r4/Logical  logical_function=AND  inputs=2  en=off  latency=0  precision=Full  arith_type=Unsigned  n_bits=8  bin_pt=2  align_bp=on  dbl_ovrd=off  block_type=logical
      settings: xl_area=[1 0 0 1 0 0 0]  block_version=VER_STRING_GOES_HERE
  PortAddress : xbsIndex_r4/Constant  const=23  gui_display_data_type=Fixed-point  arith_type=Unsigned  n_bits=8  bin_pt=0  preci_type=Single  exp_width=8  frac_width=24  explicit_period=on  period=fpgaclk  equ=P=C  opselect=C  inp2=PCIN>>17  opr=+  inp1=P  carry=CIN  dbl_ovrd=off  block_type=constant
      settings: block_version=VER_STRING_GOES_HERE
  Register1 : xbsIndex_r4/Register  init=0  rst=off  en=on  dbl_ovrd=off  block_type=register
      settings: xl_area=[4 8 0 0 0 0 0]  block_version=VER_STRING_GOES_HERE
  Relational1 : xbsIndex_r4/Relational  mode=a=b  op_type=Bool  en=off  latency=0  dbl_ovrd=off  block_type=relational
      settings: xl_area=[2 0 0 4 0 0 0]  block_version=VER_STRING_GOES_HERE
  LatchedData : Outport
  Strobe : Outport  Port=2
  wires:
  Relational1/1 -> Logical/1
  Logical/1 -> Register1/2, Strobe/1
  PortAddress/1 -> Relational1/2
  Data/1 -> Register1/1
  PortId/1 -> Relational1/1
  Write/1 -> Logical/2
  Register1/1 -> LatchedData/1

== system N3Z_tonetestError/ToneDetect/OutputRegister/Subsystem9 ==
  Data : Inport
  PortId : Inport  Port=2
  Write : Inport  Port=3
  Logical : xbsIndex_r4/Logical  logical_function=AND  inputs=2  en=off  latency=0  precision=Full  arith_type=Unsigned  n_bits=8  bin_pt=2  align_bp=on  dbl_ovrd=off  block_type=logical
      settings: xl_area=[1 0 0 1 0 0 0]  block_version=VER_STRING_GOES_HERE
  PortAddress : xbsIndex_r4/Constant  const=9  gui_display_data_type=Fixed-point  arith_type=Unsigned  n_bits=8  bin_pt=0  preci_type=Single  exp_width=8  frac_width=24  explicit_period=on  period=fpgaclk  equ=P=C  opselect=C  inp2=PCIN>>17  opr=+  inp1=P  carry=CIN  dbl_ovrd=off  block_type=constant
      settings: block_version=VER_STRING_GOES_HERE
  Register1 : xbsIndex_r4/Register  init=0  rst=off  en=on  dbl_ovrd=off  block_type=register
      settings: xl_area=[4 8 0 0 0 0 0]  block_version=VER_STRING_GOES_HERE
  Relational1 : xbsIndex_r4/Relational  mode=a=b  op_type=Bool  en=off  latency=0  dbl_ovrd=off  block_type=relational
      settings: xl_area=[2 0 0 4 0 0 0]  block_version=VER_STRING_GOES_HERE
  LatchedData : Outport
  Strobe : Outport  Port=2
  wires:
  Relational1/1 -> Logical/1
  Logical/1 -> Register1/2, Strobe/1
  PortAddress/1 -> Relational1/2
  Data/1 -> Register1/1
  PortId/1 -> Relational1/1
  Write/1 -> Logical/2
  Register1/1 -> LatchedData/1

== system N3Z_tonetestError/User_Interface/OutputRegister/Subsystem ==
  Data : Inport
  PortId : Inport  Port=2
  Write : Inport  Port=3
  Logical : xbsIndex_r4/Logical  logical_function=AND  inputs=2  en=off  latency=0  precision=Full  arith_type=Unsigned  n_bits=8  bin_pt=2  align_bp=on  dbl_ovrd=off  block_type=logical
      settings: xl_area=[1 0 0 1 0 0 0]  block_version=VER_STRING_GOES_HERE
  PortAddress : xbsIndex_r4/Constant  const=0  gui_display_data_type=Fixed-point  arith_type=Unsigned  n_bits=8  bin_pt=0  preci_type=Single  exp_width=8  frac_width=24  explicit_period=on  period=fpgaclk  equ=P=C  opselect=C  inp2=PCIN>>17  opr=+  inp1=P  carry=CIN  dbl_ovrd=off  block_type=constant
      settings: block_version=VER_STRING_GOES_HERE
  Register1 : xbsIndex_r4/Register  init=0  rst=off  en=on  dbl_ovrd=off  block_type=register
      settings: xl_area=[4 8 0 0 0 0 0]  block_version=VER_STRING_GOES_HERE
  Relational1 : xbsIndex_r4/Relational  mode=a=b  op_type=Bool  en=off  latency=0  dbl_ovrd=off  block_type=relational
      settings: xl_area=[2 0 0 4 0 0 0]  block_version=VER_STRING_GOES_HERE
  LatchedData : Outport
  Strobe : Outport  Port=2
  wires:
  Relational1/1 -> Logical/1
  Logical/1 -> Register1/2, Strobe/1
  PortAddress/1 -> Relational1/2
  Data/1 -> Register1/1
  PortId/1 -> Relational1/1
  Write/1 -> Logical/2
  Register1/1 -> LatchedData/1

== system N3Z_tonetestError/User_Interface/OutputRegister/Subsystem1 ==
  Data : Inport
  PortId : Inport  Port=2
  Write : Inport  Port=3
  Logical : xbsIndex_r4/Logical  logical_function=AND  inputs=2  en=off  latency=0  precision=Full  arith_type=Unsigned  n_bits=8  bin_pt=2  align_bp=on  dbl_ovrd=off  block_type=logical
      settings: xl_area=[1 0 0 1 0 0 0]  block_version=VER_STRING_GOES_HERE
  PortAddress : xbsIndex_r4/Constant  const=1  gui_display_data_type=Fixed-point  arith_type=Unsigned  n_bits=8  bin_pt=0  preci_type=Single  exp_width=8  frac_width=24  explicit_period=on  period=fpgaclk  equ=P=C  opselect=C  inp2=PCIN>>17  opr=+  inp1=P  carry=CIN  dbl_ovrd=off  block_type=constant
      settings: block_version=VER_STRING_GOES_HERE
  Register1 : xbsIndex_r4/Register  init=0  rst=off  en=on  dbl_ovrd=off  block_type=register
      settings: xl_area=[4 8 0 0 0 0 0]  block_version=VER_STRING_GOES_HERE
  Register2 : xbsIndex_r4/Register  init=0  rst=off  en=off  dbl_ovrd=off  block_type=register
      settings: xl_area=[1 1 0 0 0 0 0]  block_version=VER_STRING_GOES_HERE
  Register3 : xbsIndex_r4/Register  init=0  rst=off  en=off  dbl_ovrd=off  block_type=register
      settings: xl_area=[1 1 0 0 0 0 0]  block_version=VER_STRING_GOES_HERE
  Relational1 : xbsIndex_r4/Relational  mode=a=b  op_type=Bool  en=off  latency=0  dbl_ovrd=off  block_type=relational
      settings: xl_area=[2 0 0 4 0 0 0]  block_version=VER_STRING_GOES_HERE
  pulse2 : Subsystem
  LatchedData : Outport
  MemWrite : Outport  Port=2
  wires:
  Relational1/1 -> Logical/1
  Logical/1 -> Register1/2, Register3/1
  PortAddress/1 -> Relational1/2
  Data/1 -> Register1/1
  PortId/1 -> Relational1/1
  Write/1 -> Logical/2
  Register1/1 -> LatchedData/1
  Register2/1 -> pulse2/1(In1)
  Register3/1 -> Register2/1
  pulse2/1(Out1) -> MemWrite/1
